simulink model "Reforce_Experiment_FCS"  (R2021a)
settings: Solver=FixedStepDiscrete  StartTime=0.0  StopTime=Inf  FixedStep=Ts  RelTol=1e-3
PostLoadFcn:
  | , if any(exist('dsrtsu_mdlpostloadfcn', 'file') ~= 0), dsrtsu_mdlpostloadfcn('Execute', bdroot); end,
InitFcn:
  | , if any(exist('rtifpga_mdlclblib', 'file') ~= 0), rtifpga_mdlclblib('Init', bdroot); end,
model workspace (MAT data in the model file):
  FPGA_Control_Scheme_1_Buffer_1_1_1_write : Simulink.Signal (value not decoded)
  FPGA_Control_Scheme_1_Buffer_2_1_1_write : Simulink.Signal (value not decoded)
  FPGA_Control_Scheme_1_Register_1_1_1_write : Simulink.Signal (value not decoded)
  FPGA_Control_Scheme_1_Register_2_1_1_write : Simulink.Signal (value not decoded)
values from neighbouring files (symbols this model uses):
  abc2alphabeta0 = [      2/3      -1/3       -1/3 ... (first row only)    [Reforce_Init_FCS.m]
  alphabeta02abc = [  1          0 1/sqrt(2) ... (first row only)    [Reforce_Init_FCS.m]
  torque_ref_sample_lower = -torque_ref_sample_upper    (= -6.5)    [Reforce_Init_FCS.m]
  torque_ref_sample_upper = 6.5    [Reforce_Init_FCS.m]
  Ts = 50e-6    (= 5e-05)    [Reforce_Init_FCS.m]
  uf_factor = U_nom / f_nom    (= 2.82)    [Reforce_Init_FCS.m]
undefined symbols (not defined in the file or in its folder): CC, controller, init_layer_0, init_layer_1, init_layer_2, init_layer_3, init_layer_4, init_layer_5, init_layer_6, init_layer_7, init_layer_8, init_layer_9, inverter, load, motor, PLL, sensor
libraries: simulink x16, rtiproclib x13, rti1202lib_adc_class1 x8, rti1202lib_dio_class1 x4, dspfdesign x3, rtiemclib x2, rti1202lib_dac_class1 x1, embmathops x1, rti1202lib_base x1, rtitasklib x1, dsextras x1, simulink_extras x1
(part 6 of 6)

== system Reforce_Experiment_FCS/Control_Scheme/DQ_DTC/Identification_and_Safeguard/Brosch RLS/i_d_RLS/RLS/Subsystem2 ==
  reset : Inport
  xi_k : Inport  Port=2
  gamma_k-1 : Inport  Port=3
  psi_k : Inport  Port=4
  Add : Sum  Inputs=+-
  Delay1 : Delay  DelayLength=1  InitialCondition=controller.RLS.theta_0  ExternalReset=Rising
      settings: InputPortMap=u0,r5
  Product3 : Product
  Product4 : Product  Multiplication=Matrix(*)
  Sum1 : Sum  Inputs=|++
  Transpose : Math  Operator=transpose  SaturateOnIntegerOverflow=on
  theta_k : Outport
  wires:
  Delay1/1 -> Sum1/1, Product4/2  "theta_k-1"
  Product3/1 -> Sum1/2
  Product4/1 -> Add/2
  Sum1/1 -> theta_k/1, Delay1/1  "theta_k"
  Add/1 -> Product3/2
  psi_k/1 -> Add/1
  gamma_k-1/1 -> Product3/1
  Transpose/1 -> Product4/1
  xi_k/1 -> Transpose/1
  reset/1 -> Delay1/2

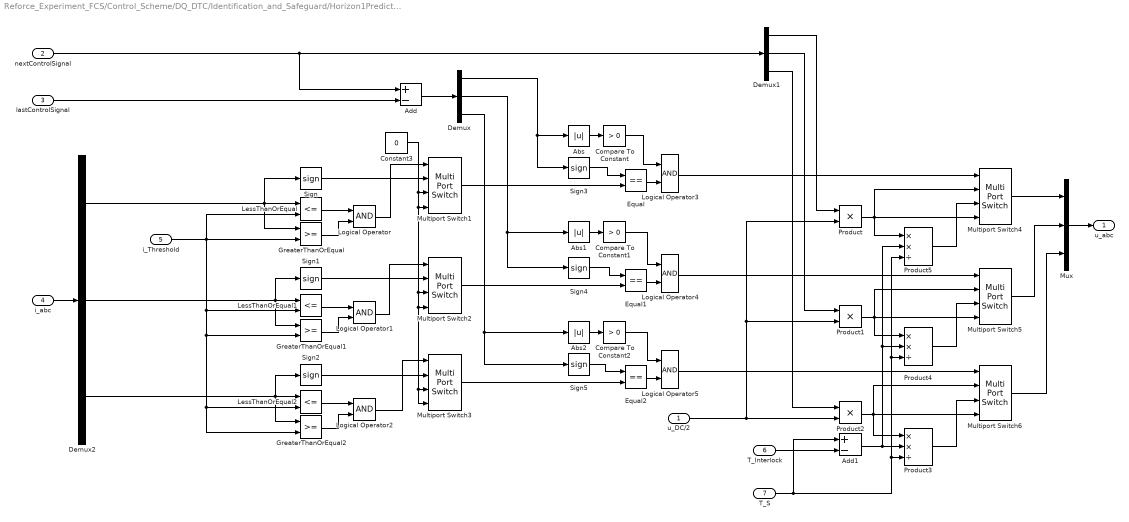
== system Reforce_Experiment_FCS/Control_Scheme/DQ_DTC/Identification_and_Safeguard/Horizon1Predictor/For Each Subsystem/VoltageApplier1/VoltageCorrection ==
  u_DC/2 : Inport
  nextControlSignal : Inport  Port=2
  lastControlSignal : Inport  Port=3
  i_abc : Inport  Port=4
  i_Threshold : Inport  Port=5
  T_Interlock : Inport  Port=6
  T_S : Inport  Port=7
  Abs : Abs
  Abs1 : Abs
  Abs2 : Abs
  Add : Sum  Inputs=+-
  Add1 : Sum  Inputs=+-
  Compare To Constant : simulink/Logic and Bit Operations/Compare To Constant  relop=>  const=0  OutDataTypeStr=boolean
  Compare To Constant1 : simulink/Logic and Bit Operations/Compare To Constant  relop=>  const=0  OutDataTypeStr=boolean
  Compare To Constant2 : simulink/Logic and Bit Operations/Compare To Constant  relop=>  const=0  OutDataTypeStr=boolean
  Constant3 : Constant  Value=0
  Demux : Demux  Outputs=3
  Demux1 : Demux  Outputs=3
  Demux2 : Demux  Outputs=3
  Equal : RelationalOperator  Operator===  OutDataTypeStr=boolean  RndMeth=Simplest
  Equal1 : RelationalOperator  Operator===  OutDataTypeStr=boolean  RndMeth=Simplest
  Equal2 : RelationalOperator  Operator===  OutDataTypeStr=boolean  RndMeth=Simplest
  GreaterThanOrEqual : RelationalOperator  OutDataTypeStr=boolean  RndMeth=Simplest
  GreaterThanOrEqual1 : RelationalOperator  OutDataTypeStr=boolean  RndMeth=Simplest
  GreaterThanOrEqual2 : RelationalOperator  OutDataTypeStr=boolean  RndMeth=Simplest
  LessThanOrEqual : RelationalOperator  Operator=<=  OutDataTypeStr=boolean  RndMeth=Simplest
  LessThanOrEqual1 : RelationalOperator  Operator=<=  OutDataTypeStr=boolean  RndMeth=Simplest
  LessThanOrEqual2 : RelationalOperator  Operator=<=  OutDataTypeStr=boolean  RndMeth=Simplest
  Logical Operator{,1..5} (6 alike) : Logic  AllPortsSameDT=off  OutDataTypeStr=boolean
  Multiport Switch{1..6} (6 alike) : MultiPortSwitch  DataPortOrder=Specify indices  DataPortIndices={0,1}  DataPortForDefault=Additional data port
  Mux : Mux  Inputs=3
  Product : Product
  Product1 : Product
  Product2 : Product
  Product3 : Product  Inputs=**/
  Product4 : Product  Inputs=**/
  Product5 : Product  Inputs=**/
  Sign{,1..5} (6 alike) : Signum
  u_abc : Outport
  wires:
  GreaterThanOrEqual2/1 -> Logical Operator2/2
  Constant3/1 -> Multiport Switch3/4, Multiport Switch3/3, Multiport Switch2/4, Multiport Switch2/3, Multiport Switch1/4, Multiport Switch1/3
  Demux2/1 -> GreaterThanOrEqual/1, Sign/1, LessThanOrEqual/1
  u_DC/2/1 -> Product/2, Product1/2, Product2/2
  T_S/1 -> Product5/3, Product4/3, Product3/3, Add1/1
  Demux/1 -> Sign3/1, Abs/1
  GreaterThanOrEqual1/1 -> Logical Operator1/2
  LessThanOrEqual/1 -> Logical Operator/1
  Add/1 -> Demux/1
  LessThanOrEqual1/1 -> Logical Operator1/1
  Abs2/1 -> Compare To Constant2/1
  Abs/1 -> Compare To Constant/1
  i_Threshold/1 -> LessThanOrEqual/2, GreaterThanOrEqual2/2, LessThanOrEqual2/2, GreaterThanOrEqual1/2, LessThanOrEqual1/2, GreaterThanOrEqual/2
  Product/1 -> Product5/1, Multiport Switch4/4, Multiport Switch4/2
  Add1/1 -> Product4/2, Product5/2, Product3/2
  Abs1/1 -> Compare To Constant1/1
  Multiport Switch6/1 -> Mux/3
  Demux1/2 -> Product1/1
  Multiport Switch1/1 -> Equal/2
  Multiport Switch5/1 -> Mux/2
  Product4/1 -> Multiport Switch5/3
  T_Interlock/1 -> Add1/2
  Logical Operator1/1 -> Multiport Switch2/1
  Logical Operator/1 -> Multiport Switch1/1
  GreaterThanOrEqual/1 -> Logical Operator/2
  nextControlSignal/1 -> Add/1, Demux1/1
  Compare To Constant1/1 -> Logical Operator4/1
  Demux1/1 -> Product/1
  Demux1/3 -> Product2/1
  Logical Operator4/1 -> Multiport Switch5/1
  Product5/1 -> Multiport Switch4/3
  Product1/1 -> Product4/1, Multiport Switch5/4, Multiport Switch5/2
  Logical Operator2/1 -> Multiport Switch3/1
  lastControlSignal/1 -> Add/2
  Compare To Constant/1 -> Logical Operator3/1
  Product2/1 -> Product3/1, Multiport Switch6/4, Multiport Switch6/2
  LessThanOrEqual2/1 -> Logical Operator2/1
  Sign/1 -> Multiport Switch1/2
  Product3/1 -> Multiport Switch6/3
  Logical Operator3/1 -> Multiport Switch4/1
  Sign1/1 -> Multiport Switch2/2
  Sign2/1 -> Multiport Switch3/2
  Logical Operator5/1 -> Multiport Switch6/1
  Compare To Constant2/1 -> Logical Operator5/1
  Multiport Switch4/1 -> Mux/1
  Demux2/2 -> Sign1/1, GreaterThanOrEqual1/1, LessThanOrEqual1/1
  Demux2/3 -> Sign2/1, GreaterThanOrEqual2/1, LessThanOrEqual2/1
  Equal/1 -> Logical Operator3/2
  Sign3/1 -> Equal/1
  Sign4/1 -> Equal1/1
  Multiport Switch2/1 -> Equal1/2
  Demux/2 -> Abs1/1, Sign4/1
  Equal1/1 -> Logical Operator4/2
  Demux/3 -> Sign5/1, Abs2/1
  Multiport Switch3/1 -> Equal2/2
  Sign5/1 -> Equal2/1
  Equal2/1 -> Logical Operator5/2
  Mux/1 -> u_abc/1
  i_abc/1 -> Demux2/1

== system Reforce_Experiment_FCS/Control_Scheme/DQ_DTC/Identification_and_Safeguard/Horizon1Predictor/For Each Subsystem/VoltageApplier1/abc2dq1 ==
  abc : Inport
  epsilon : Inport  Port=2
  Gain1 : Gain  Gain=abc2alphabeta0  Multiplication=Matrix(K*u)
  alphabeta02dq : Subsystem
  dq : Outport
  wires:
  alphabeta02dq/1(dq) -> dq/1
  abc/1 -> Gain1/1
  Gain1/1 -> alphabeta02dq/1(alphabeta0)
  epsilon/1 -> alphabeta02dq/2(epsilon)

== system Reforce_Experiment_FCS/Control_Scheme/DQ_DTC/Identification_and_Safeguard/Horizon1Predictor/For Each Subsystem/VoltageApplier1/abc2dq1/alphabeta02dq ==
  alphabeta0 : Inport
  epsilon : Inport  Port=2
  Cos : Trigonometry  Operator=cos  NumberOfDataPoints=64
  Demux : Demux  Outputs=3
  Gain1 : Gain  Gain=-1
  Gain2 : Gain  Gain=-1
  Mux : Mux  Inputs=2
  Product{,1..3} (4 alike) : Product
  Sin : Trigonometry  NumberOfDataPoints=64
  Sum : Sum  Inputs=|++
  Sum1 : Sum  Inputs=|++
  Terminator : Terminator
  dq : Outport
  wires:
  Gain2/1 -> Cos/1, Sin/1
  Product3/1 -> Sum1/2
  Sin/1 -> Product2/2, Gain1/1
  Product2/1 -> Sum1/1
  Product/1 -> Sum/2
  Gain1/1 -> Product/2
  Demux/2 -> Product/1, Product3/1
  Product1/1 -> Sum/1
  Cos/1 -> Product3/2, Product1/2
  Demux/1 -> Product2/1, Product1/1
  Mux/1 -> dq/1
  Sum1/1 -> Mux/2
  Sum/1 -> Mux/1
  Demux/3 -> Terminator/1
  alphabeta0/1 -> Demux/1
  epsilon/1 -> Gain2/1

== matlab function Reforce_Experiment_FCS/Control_Scheme/DQ_DTC/Identification_and_Safeguard/ABE_d_LUT ==
  data: w_me input; A_d output; i_dq input; B_d output; E_d output; controller parameter; motor parameter; Ts parameter
function [A_d, B_d, E_d] = fcn(w_me, i_dq, controller, motor, Ts)

L_dd = LUT2D(controller.preindl.LUT.x_vec,controller.preindl.LUT.y_vec,controller.preindl.LUT.L_dd_map,i_dq(1),i_dq(2));
L_qq = LUT2D(controller.preindl.LUT.x_vec,controller.preindl.LUT.y_vec,controller.preindl.LUT.L_qq_map,i_dq(1),i_dq(2));
L_dq = LUT2D(controller.preindl.LUT.x_vec,controller.preindl.LUT.y_vec,controller.preindl.LUT.L_dq_map,i_dq(1),i_dq(2));
L_qd = LUT2D(controller.preindl.LUT.x_vec,controller.preindl.LUT.y_vec,controller.preindl.LUT.L_qd_map,i_dq(1),i_dq(2));

Psi_d = LUT2D(controller.preindl.LUT.x_vec,controller.preindl.LUT.y_vec,controller.preindl.LUT.Psi_d_map,i_dq(1),i_dq(2));
Psi_q = LUT2D(controller.preindl.LUT.x_vec,controller.preindl.LUT.y_vec,controller.preindl.LUT.Psi_q_map,i_dq(1),i_dq(2)); 


w_el = motor.param.p * w_me;
inv_L = 1 / (L_dd * L_qq - L_dq * L_qd) * [L_qq -L_dq;
                                          -L_qd  L_dd];


A_d = eye(2) - Ts * inv_L * motor.param.R_s;

B_d = Ts * inv_L;

E_d = - Ts * w_el * inv_L * [-Psi_q;
                              Psi_d;];

== matlab function Reforce_Experiment_FCS/Control_Scheme/current_FOC_v1_2/Begrenzung des Raumzeigers ==
  data: U_d input; U_d_limit output; U_q input; I_q input; U_q_limit output; U_ZK input; limit_on output; Fehler output; Fall output


function [U_d_limit, U_q_limit, limit_on, Fehler, Fall] = fcn(U_d, U_q, I_q, U_ZK)
%#codegen

% maximale Amplitude des Raumzeigers bzw. der Leiterspannung
   % ohne Addition einer 3ten Harmonischen   U^_LN = U_ZK/2;
   U_RZ_max = (U_ZK*0.5);
   %bei Offsetaddition der 3te Harmonischen  U^_LN = U_ZK/sqrt(3);
   % U_RZ_max = U_ZK/sqrt(3);

% Betrag des Raumzeigers aus U_d und U_q
U_RZ_betrag = sqrt(U_d^2 + U_q^2);

% Ist eine Begrenzung notwendig?
if ( U_RZ_betrag > U_RZ_max )   
    limit_on = 1;
% Begrenzung notwendig -> motorischer oder generatorischer Betrieb?
    if ( (U_d<0) && (sign(U_q)==sign(I_q)) ) % Motorbetrieb
       
        Fehler = 0;
        if ( abs(U_d) > 0.95*U_RZ_max )
        %true
        U_d_limit = sign(U_d)*0.95*U_RZ_max;
        U_q_limit = sign(U_q)*sqrt(U_RZ_max^2-U_d_limit^2);
        Fall = 2;
        else
        %false
        U_d_limit = U_d;
        U_q_limit = sign(U_q)*sqrt(U_RZ_max^2-U_d_limit^2);
        Fall = 1;
        end    
    
    
    elseif ( (U_d>0) && (sign(U_q)~=sign(I_q)) ) % Generatorbetrieb
    
        Fehler = 0;
        if ( abs(U_q) > 0.95*U_RZ_max )
        %true
        U_q_limit = sign(U_q)*0.95*U_RZ_max;
        U_d_limit = sign(U_d)*sqrt(U_RZ_max^2-U_q_limit^2);
        Fall = 4;
        
        else 
        % false
        U_q_limit = U_q;
        U_d_limit = sign(U_d)*sqrt(U_RZ_max^2-U_q_limit^2);
        Fall = 3;
        end
        
    else % Weder motorischer noch generatorischer Betrieb => Fehler 
    U_d_limit = U_d;
    U_q_limit = U_q;
    Fehler = 1;
    Fall = 5;
    end
    
else
% keine Begrenzung notwendig
    U_d_limit = U_d;
    U_q_limit = U_q;
    limit_on = 0;
    Fehler = 0;
    Fall = 0;
end

== matlab function Reforce_Experiment_FCS/Control_Scheme/DQ_DTC/Action_Processing/EpsilonSafetyActionSelection_old ==
  settings: updateMethod=DISCRETE
  data: argmax_Q input; a_out output int32; a_policy output; a_allowed input; a_current input; epsilon input; safeguard_active output; controller parameter
function [a_out, a_policy, safeguard_active]= fcn(argmax_Q, a_allowed, a_current, epsilon, controller)

a_allowed = a_allowed(~isnan(a_allowed));
safeguard_active = 1;

if rand < epsilon
    % determine action from momentary policy
    a_policy = int32(randi(controller.DQDTC.action_dim))-1;
else
    a_policy = argmax_Q;
end

if isempty(a_allowed)
    % if no action can comply with the op.limits, 
    % apply action that minimizes current
    [~, I] = min(a_current); % argmin
    a_out = int32(I-1);
else
    if ismember(a_policy, a_allowed)
        % apply action that is optimal according to DQN
        a_out = a_policy;  
        safeguard_active = 0;
    else
        % if policy action does not comply with op.limits, apply random
        % action that does
        random_index = randi(length(a_allowed));
        a_out = int32(a_allowed(random_index));
    end
end

== matlab function Reforce_Experiment_FCS/Control_Scheme/DQ_DTC/Learning_Rate_Schedule ==
  data: time input; lr output; controller parameter; epsilon output
function [lr, epsilon] = fcn(time, controller)

alpha = time / controller.DQDTC.schedule_time;

lr = (1-alpha) * controller.DQDTC.initial_lr + alpha * controller.DQDTC.final_lr;
epsilon = (1-alpha) * controller.DQDTC.initial_epsilon + alpha * controller.DQDTC.final_epsilon;

if time >= controller.DQDTC.schedule_time
    lr = controller.DQDTC.final_lr;
    epsilon = controller.DQDTC.final_epsilon;
end

== matlab function Reforce_Experiment_FCS/Control_Scheme/PreindlMPC/Preindls_Cost ==
  data: i_dq_all input; cost output; w_el input; T_ref input; u_dc input; lambda_current input; lambda_limit input; physical_parameters input; motor parameter; controller parameter
function cost = fcn(i_dq_all, w_el, T_ref, u_dc, lambda_current, lambda_limit, physical_parameters, motor, controller)

p = motor.param.p;

i_nom = motor.nominal.i;
zeta = controller.preindl.zeta;
psi_p = controller.preindl.LUT.psi_p;

%psi_p = physical_parameters(2);
l_d = physical_parameters(3);
l_q = physical_parameters(4);
delta_l = physical_parameters(5);
frac_l_dq = physical_parameters(6);
frac_l_qd = 1 / frac_l_dq;

cost = zeros(8,1);
for i=1:8
idx = 2*i;

i_dq = i_dq_all(idx-1:idx);
i_d2 = i_dq(1)^2;
i_q2 = i_dq(2)^2;

T_pred = 1.5 * p * (psi_p + delta_l * i_dq(1)) * i_dq(2);
c_torque = (T_ref - T_pred)^2;


c_current1 = (i_dq(1) + delta_l / psi_p * (i_d2 - i_q2))^2;
c_limit1 = i_nom - sqrt(i_d2 + i_q2);
if c_limit1 > 0
    c_limit1 = 0;
else
    c_limit1 = c_limit1^2;
end

c_limit2 = 2 * delta_l / psi_p * i_dq(1) + 1;
if c_limit2 > 0
    c_limit2 = 0;
else
    c_limit2 = c_limit2^2;
end

xi = sqrt((l_q * i_dq(2))^2 + (l_d * i_dq(1) + psi_p)^2) - zeta * u_dc / sqrt(3) / (abs(w_el) + eps);
c_limit3 = 0;
if xi < 0
    c_limit3 = xi^2;
end

theta = psi_p^2 / l_q + psi_p * (2 * frac_l_dq - 1) * i_dq(1) + l_d * (frac_l_dq - 1) * i_d2 + l_q * (frac_l_qd - 1) * i_q2;
c_limit4 = 0;
if theta < 0
    c_limit4 = theta^2;
end

i_d_MPTC = - psi_p / 2 - sqrt((psi_p / 2)^2 + delta_l^2 * i_q2);
if i_d_MPTC > delta_l * i_dq(1)
    left_MTPC = 1;
else
    left_MTPC = 0;
end

c_current2 = (sqrt((frac_l_qd * i_dq(2))^2 + (i_dq(1) + psi_p / l_d)^2) - zeta * u_dc / sqrt(3) / (abs(w_el) + eps) / l_d)^2;

if c_current2 < c_current1 && left_MTPC && abs(w_el) > controller.preindl.w_boundary
    c_current = c_current2;
else
    c_current = c_current1;
end  

if abs(w_el) > controller.preindl.w_boundary
    cost(i) = c_torque + lambda_current * c_current + lambda_limit * (c_limit1 + c_limit2 + c_limit3 + c_limit4);
else
    cost(i) = c_torque + lambda_current * c_current + lambda_limit * (c_limit1 + c_limit2);
end
end

== matlab function Reforce_Experiment_FCS/Control_Scheme/MATLAB Function1 ==
  data: HotButton input; y output; schedulerClock input; stop input
function y = fcn(HotButton, schedulerClock, stop)
persistent learning block_start
if isempty(learning)
    learning = false;
    block_start = false;
end

if HotButton && not((schedulerClock == 0.0) || stop) && not(block_start)
    learning = true;
elseif (schedulerClock == 0.0) || stop
    learning = false;
    block_start = true;
end

if not(stop) && not(HotButton)
    block_start = false;
end

y = learning;

== stateflow chart Reforce_Experiment_FCS/Control_Scheme/Chart ==
  state Waiting
    entry:
    idx = 0;
    T_out = 0;
    exit:
    idx = idx + 1;
  state Active
    entry:
    T_out = T_ref(idx);
    exit:
    idx = idx + 1;
  (default) -> Waiting
  (junction 14) -> Waiting [order 1] : [idx >= length(T_ref)]
  Waiting -> Active : [activate]
  Active -> (junction 14) : [after(0.5, sec)]
  (junction 14) -> Active [order 2]
  data: activate input; T_out output; idx local; T_ref parameter

== matlab function Reforce_Experiment_FCS/Control_Scheme/DQ_DTC/Action_Processing/EpsilonSafetyActionSelection ==
  settings: updateMethod=DISCRETE
  data: Q_values input; a_out output int32; a_policy output; a_allowed input; a_current input; epsilon input; safeguard_active output
function [a_out, a_policy, safeguard_active]= fcn(Q_values, a_allowed, a_current, epsilon)

a_allowed = a_allowed(~isnan(a_allowed));
safeguard_active = 1;

if rand < epsilon
    % determine action from momentary policy
    a_policy = int32(randi(length(Q_values))-1);

    if ismember(a_policy, a_allowed)
        a_out = a_policy;
        safeguard_active = 0;
    else
        if isempty(a_allowed)
            [~, I] = min(a_current); % argmin
            a_out = int32(I-1);
        else
            random_index = randi(length(a_allowed));    
            a_out = int32(a_allowed(random_index));
        end
    end

else
    [~, I] = max(Q_values);
    a_policy = int32(I-1);

    if ismember(a_policy, a_allowed)
        a_out = a_policy;
        safeguard_active = 0;
    else
        if isempty(a_allowed)
            [~, I] = min(a_current); % argmin
            a_out = int32(I-1);
        else
            [~, I] = max(Q_values(a_allowed+1));
            a_out = int32(a_allowed(I));
        end
    end       
end

== matlab function Reforce_Experiment_FCS/Control_Scheme/MATLAB Function ==
  data: u_DC input; chop output; chop_low input; chop_high input; chop_last input
function chop = fcn(u_DC, chop_low, chop_high, chop_last)

%% for PWM chopping

chop = (u_DC - chop_low) / (chop_high - chop_low);

if chop > 1.0
    chop = 1.0;
end

if chop < 0.0
    chop = 0.0;
end


%% for non-PWM chopping
% if u_DC > chop_high
%     chop = true;
% elseif u_DC < chop_low
%     chop = false;
% else
%     chop = chop_last;
end
